simulink model "valve_map"  (R2024b)
settings: Solver=FixedStepDiscrete  StartTime=0.0  StopTime=300  FixedStep=dev.dt  RelTol=1e-3
undefined symbols (not defined in the file or in its folder): disfilt, dspblkCoreblockFVToolHelper, dt, gcbh
libraries: simulink x1, subsignallib x1
settings Model: SimulationMode=external  ExtModeEnableFloating=off  ExtModeTrigDuration=100000  Creator=pro  LastModifiedBy=af49v
settings SolverCC: ConcurrentTasks=on  AlgebraicLoopSolver=TrustRegion  PositivePriorityOrder=on  AutoInsertRateTranBlk=on
settings DataIOCC: MaxDataPoints=500  SaveOutput=off  DSMLogging=off  SaveTime=off  ReturnWorkspaceOutputs=off
settings OptimizationCC: BlockReduction=off  OptimizeBlockIOStorage=off  EnhancedBackFolding=on  PassReuseOutputArgsThreshold=0  MaxStackSize=64  OptimizeBlockOrder=speed  DifferentSizesBufferReuse=on
settings DebuggingCC: AlgebraicLoopMsg=error  TasksWithSamePriorityMsg=none  IntegerOverflowMsg=error  ParameterUnderflowMsg=error  ParameterTunabilityLossMsg=error  UnconnectedInputMsg=warning  UnconnectedOutputMsg=warning  UnconnectedLineMsg=warning  AllowSymbolicDim=off  NonBusSignalsTreatedAsBus=error  SFInvalidInputDataAccessInChartInitDiag=error
settings HardwareCC: ProdBitPerLong=64  ProdLongLongMode=on  ProdHWDeviceType=Intel->x86-64 (Linux 64)  HardwareBoardFeatureSet=SoCBlockset
settings ModelReferenceCC: EnableRefExpFcnMdlSchedulingChecks=on
settings SFSimCC: MATLABDynamicMemAlloc=off
settings RTWCC: Description=Speedgoat Real-Time Target Machine  SystemTargetFile=speedgoat.tlc  TemplateMakefile=slrealtime_default_tmf  RTWVerbose=off  Toolchain=Simulink Real-Time Toolchain  BuildConfiguration=Faster Runs  CodeExecutionProfiling=on  TargetLang=C++  GPUComputeCapability=3.5  DLArmComputeVersion=19.05
settings CodeAppCC: ForceParamTrailComments=on  OperatorAnnotations=on
settings SimulinkRealTimeTargetCC: InstructionSetFMA=off  LogToMDFFile=off

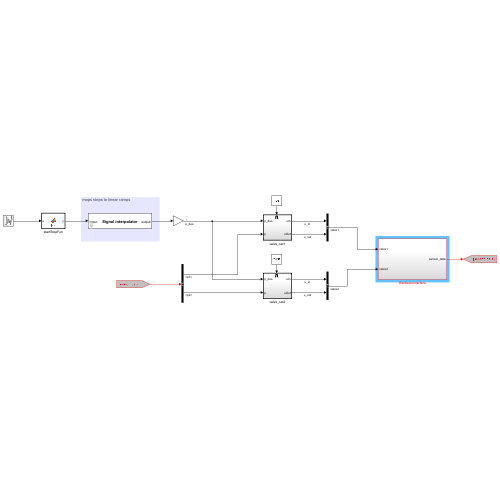
[thumbnail: Simulink's stored preview of the top-level diagram]
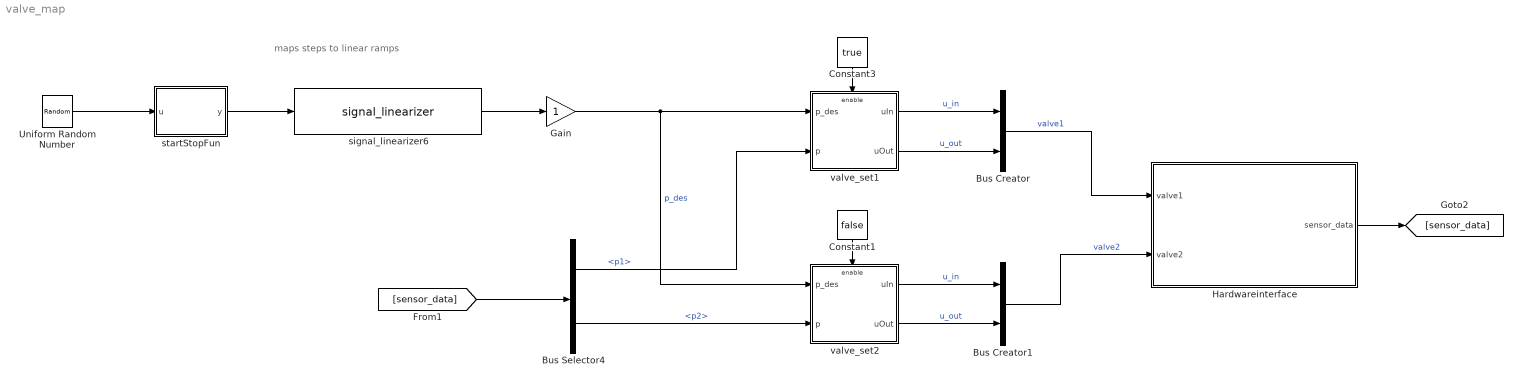
== system valve_map ==
  note: maps steps to linear ramps
  Bus Creator : BusCreator  Inputs=2
  Bus Creator1 : BusCreator  Inputs=2
  Bus Selector4 : BusSelector  OutputSignals=p1,p2
  Constant1 : Constant  Value=false
  Constant3 : Constant  Value=true
  Gain : Gain
  Hardwareinterface : Subsystem
  Uniform Random Number : UniformRandomNumber  Minimum=-0.5  Maximum=6.5  SampleTime=dt
  signal_linearizer6 : subsignallib/signal_linearizer  param_low=1  param_high=dt  es_filt_enabled=on  es_ts=4
      settings: SourceProductName=Signals
  startStopFun : MATLAB Function  TreatAsAtomicUnit=on
  valve_set1 : Subsystem
  valve_set2 : Subsystem
  wires:
  Bus Selector4/1 -> valve_set1/2(p)  "<p1>"
  Gain/1 -> valve_set1/1(p_des), valve_set2/1(p_des)  "p_des"
  Bus Selector4/2 -> valve_set2/2(p)  "<p2>"
  valve_set1/2(uOut) -> Bus Creator/2  "u_out"
  Constant1/1 -> valve_set2/Enable
  Constant3/1 -> valve_set1/Enable
  startStopFun/1(y) -> signal_linearizer6/1
  signal_linearizer6/1 -> Gain/1
  Uniform Random Number/1 -> startStopFun/1(u)
  valve_set2/1(uIn) -> Bus Creator1/1  "u_in"
  valve_set1/1(uIn) -> Bus Creator/1  "u_in"
  [sensor_data] -> Bus Selector4/1
  Bus Creator1/1 -> Hardwareinterface/2(valve2)  "valve2"
  Bus Creator/1 -> Hardwareinterface/1(valve1)  "valve1"
  Hardwareinterface/1(sensor_data) -> [sensor_data]
  valve_set2/2(uOut) -> Bus Creator1/2  "u_out"

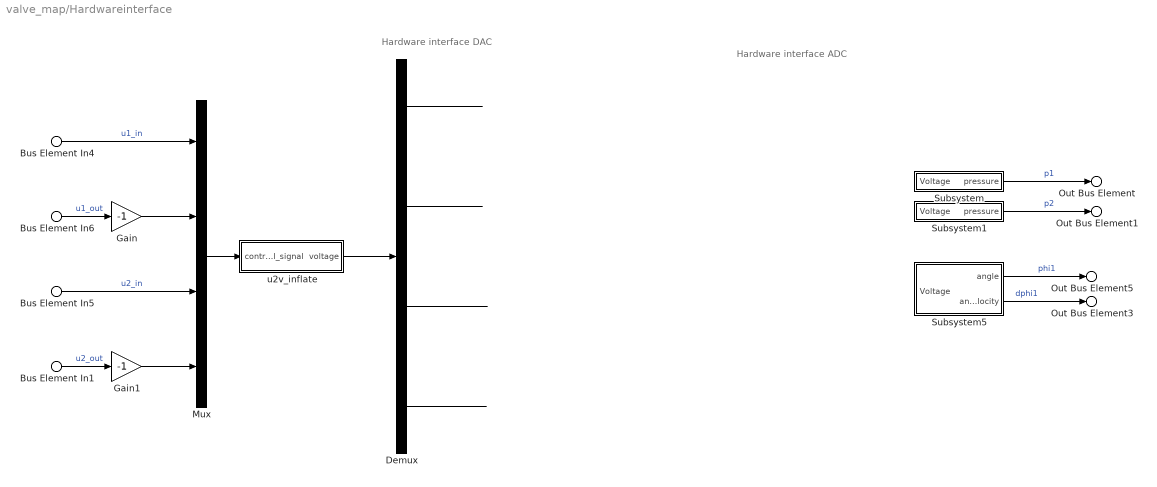
== system valve_map/Hardwareinterface ==
  note: Hardware interface ADC
  note: Hardware interface DAC
  Bus Element In4 : Inport  PortName=valve1  Element=u_in
  Bus Element In6 : Inport  PortName=valve1  Element=u_out
  Bus Element In5 : Inport  Port=2  PortName=valve2  Element=u_in
  Bus Element In1 : Inport  Port=2  PortName=valve2  Element=u_out
  Demux : Demux
  Gain : Gain  Gain=-1
  Gain1 : Gain  Gain=-1
  Mux : Mux
  Subsystem : Subsystem
  Subsystem1 : Subsystem
  Subsystem5 : Subsystem
  u2v_inflate : Subsystem
  Out Bus Element : Outport  PortName=sensor_data  Element=p1
  Out Bus Element1 : Outport  PortName=sensor_data  Element=p2
  Out Bus Element5 : Outport  PortName=sensor_data  Element=phi1
  Out Bus Element3 : Outport  PortName=sensor_data  Element=dphi1
  wires:
  Subsystem/1(pressure) -> Out Bus Element/1  "p1"
  ? -> Subsystem/1(Voltage)
  ? -> Subsystem1/1(Voltage)
  Subsystem1/1(pressure) -> Out Bus Element1/1  "p2"
  Bus Element In4/1 -> Mux/1  "u1_in"
  ? -> Subsystem5/1(Voltage)
  Subsystem5/1(angle) -> Out Bus Element5/1  "phi1"
  Bus Element In6/1 -> Gain/1  "u1_out"
  Gain/1 -> Mux/2
  Bus Element In5/1 -> Mux/3  "u2_in"
  Bus Element In1/1 -> Gain1/1  "u2_out"
  Gain1/1 -> Mux/4
  Subsystem5/2(angle velocity) -> Out Bus Element3/1  "dphi1"
  Mux/1 -> u2v_inflate/1(control_signal)
  u2v_inflate/1(voltage) -> Demux/1
  Demux/1 -> ?
  Demux/2 -> ?
  Demux/3 -> ?
  Demux/4 -> ?

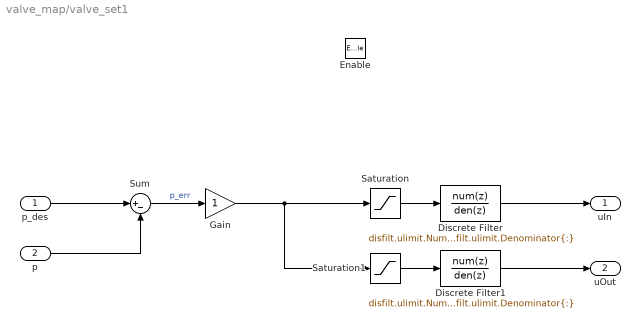
== system valve_map/valve_set1 ==
  p_des : Inport
  p : Inport  Port=2
  Enable : EnablePort
  Discrete Filter : DiscreteFilter  LoadFcn=dspblkCoreblockFVToolHelper(gcbh,'load');  Numerator=disfilt.ulimit.Numerator{:}  Denominator=disfilt.ulimit.Denominator{:}  InitialStates=0.2
      settings: CopyFcn=dspblkCoreblockFVToolHelper(gcbh,'copy');  DeleteFcn=dspblkCoreblockFVToolHelper(gcbh,'close');  ModelCloseFcn=dspblkCoreblockFVToolHelper(gcbh,'close');  PreSaveFcn=dspblkCoreblockFVToolHelper(gcbh,'presave');  PostSaveFcn=dspblkCoreblockFVToolHelper(gcbh,'postsave');  CloseFcn=dspblkCoreblockFVToolHelper(gcbh,'close');
  Discrete Filter1 : DiscreteFilter  LoadFcn=dspblkCoreblockFVToolHelper(gcbh,'load');  Numerator=disfilt.ulimit.Numerator{:}  Denominator=disfilt.ulimit.Denominator{:}  InitialStates=-0.2
      settings: CopyFcn=dspblkCoreblockFVToolHelper(gcbh,'copy');  DeleteFcn=dspblkCoreblockFVToolHelper(gcbh,'close');  ModelCloseFcn=dspblkCoreblockFVToolHelper(gcbh,'close');  PreSaveFcn=dspblkCoreblockFVToolHelper(gcbh,'presave');  PostSaveFcn=dspblkCoreblockFVToolHelper(gcbh,'postsave');  CloseFcn=dspblkCoreblockFVToolHelper(gcbh,'close');
  Gain : Gain
  Saturation : Saturate  UpperLimit=1  LowerLimit=0
  Saturation1 : Saturate  UpperLimit=0  LowerLimit=-1
  Sum : Sum  Inputs=|+-
  uIn : Outport  OutputWhenDisabled=reset  InitialOutput=0
  uOut : Outport  Port=2  OutputWhenDisabled=reset  InitialOutput=0
  wires:
  Gain/1 -> Saturation/1, Saturation1/1
  Sum/1 -> Gain/1  "p_err"
  p/1 -> Sum/2
  p_des/1 -> Sum/1
  Saturation1/1 -> Discrete Filter1/1
  Saturation/1 -> Discrete Filter/1
  Discrete Filter/1 -> uIn/1
  Discrete Filter1/1 -> uOut/1

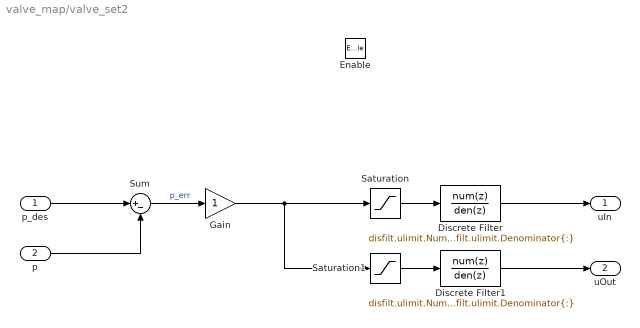
== system valve_map/valve_set2 ==
  p_des : Inport
  p : Inport  Port=2
  Enable : EnablePort
  Discrete Filter : DiscreteFilter  LoadFcn=dspblkCoreblockFVToolHelper(gcbh,'load');  Numerator=disfilt.ulimit.Numerator{:}  Denominator=disfilt.ulimit.Denominator{:}  InitialStates=0.2
      settings: CopyFcn=dspblkCoreblockFVToolHelper(gcbh,'copy');  DeleteFcn=dspblkCoreblockFVToolHelper(gcbh,'close');  ModelCloseFcn=dspblkCoreblockFVToolHelper(gcbh,'close');  PreSaveFcn=dspblkCoreblockFVToolHelper(gcbh,'presave');  PostSaveFcn=dspblkCoreblockFVToolHelper(gcbh,'postsave');  CloseFcn=dspblkCoreblockFVToolHelper(gcbh,'close');
  Discrete Filter1 : DiscreteFilter  LoadFcn=dspblkCoreblockFVToolHelper(gcbh,'load');  Numerator=disfilt.ulimit.Numerator{:}  Denominator=disfilt.ulimit.Denominator{:}  InitialStates=-0.2
      settings: CopyFcn=dspblkCoreblockFVToolHelper(gcbh,'copy');  DeleteFcn=dspblkCoreblockFVToolHelper(gcbh,'close');  ModelCloseFcn=dspblkCoreblockFVToolHelper(gcbh,'close');  PreSaveFcn=dspblkCoreblockFVToolHelper(gcbh,'presave');  PostSaveFcn=dspblkCoreblockFVToolHelper(gcbh,'postsave');  CloseFcn=dspblkCoreblockFVToolHelper(gcbh,'close');
  Gain : Gain
  Saturation : Saturate  UpperLimit=1  LowerLimit=0
  Saturation1 : Saturate  UpperLimit=0  LowerLimit=-1
  Sum : Sum  Inputs=|+-
  uIn : Outport  OutputWhenDisabled=reset  InitialOutput=0
  uOut : Outport  Port=2  OutputWhenDisabled=reset  InitialOutput=0
  wires:
  Gain/1 -> Saturation/1, Saturation1/1
  Sum/1 -> Gain/1  "p_err"
  p/1 -> Sum/2
  p_des/1 -> Sum/1
  Saturation1/1 -> Discrete Filter1/1
  Saturation/1 -> Discrete Filter/1
  Discrete Filter/1 -> uIn/1
  Discrete Filter1/1 -> uOut/1

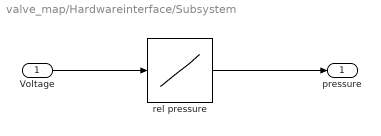
== system valve_map/Hardwareinterface/Subsystem ==
  Voltage : Inport
  rel pressure : Lookup_n-D  NumberOfTableDimensions=1  BreakpointsForDimension1=[0 10]  Table=[0 10]  InternalRulePriority=Speed  RndMeth=Simplest
  pressure : Outport  VectorParamsAs1DForOutWhenUnconnected=off
  wires:
  Voltage/1 -> rel pressure/1
  rel pressure/1 -> pressure/1

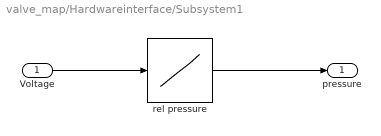
== system valve_map/Hardwareinterface/Subsystem1 ==
  Voltage : Inport
  rel pressure : Lookup_n-D  NumberOfTableDimensions=1  BreakpointsForDimension1=[0 10]  Table=[0 10]  InternalRulePriority=Speed  RndMeth=Simplest
  pressure : Outport  VectorParamsAs1DForOutWhenUnconnected=off
  wires:
  Voltage/1 -> rel pressure/1
  rel pressure/1 -> pressure/1

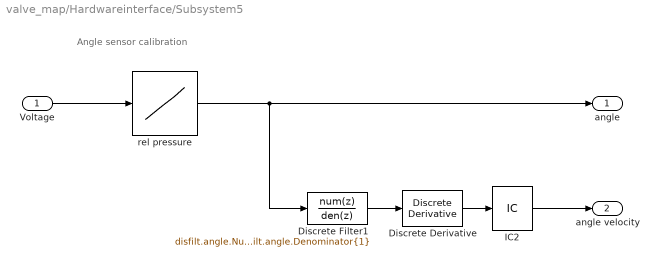
== system valve_map/Hardwareinterface/Subsystem5 ==
  note: Angle sensor calibration
  Voltage : Inport
  Discrete Derivative : simulink/Discrete/Discrete Derivative  gainval=1.0  ICPrevScaledInput=0.0  OutMin=[]  OutMax=[]  OutDataType=fixdt(1, 16)  OutScaling=2^-10  DoSatur=off
  Discrete Filter1 : DiscreteFilter  LoadFcn=dspblkCoreblockFVToolHelper(gcbh,'load');  Numerator=disfilt.angle.Numerator{1}  Denominator=disfilt.angle.Denominator{1}
      settings: CopyFcn=dspblkCoreblockFVToolHelper(gcbh,'copy');  DeleteFcn=dspblkCoreblockFVToolHelper(gcbh,'close');  ModelCloseFcn=dspblkCoreblockFVToolHelper(gcbh,'close');  PreSaveFcn=dspblkCoreblockFVToolHelper(gcbh,'presave');  PostSaveFcn=dspblkCoreblockFVToolHelper(gcbh,'postsave');  CloseFcn=dspblkCoreblockFVToolHelper(gcbh,'close');
  IC2 : InitialCondition
  rel pressure : Lookup_n-D  NumberOfTableDimensions=1  BreakpointsForDimension1=[2.167 3.14]  Table=[0.7854 -0.7854]  InternalRulePriority=Speed  RndMeth=Simplest
  angle : Outport  VectorParamsAs1DForOutWhenUnconnected=off
  angle velocity : Outport  Port=2  VectorParamsAs1DForOutWhenUnconnected=off
  wires:
  Discrete Derivative/1 -> IC2/1
  IC2/1 -> angle velocity/1
  rel pressure/1 -> angle/1, Discrete Filter1/1
  Discrete Filter1/1 -> Discrete Derivative/1
  Voltage/1 -> rel pressure/1

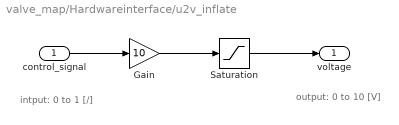
== system valve_map/Hardwareinterface/u2v_inflate ==
  note: intput: 0 to 1 [/]
  note: output: 0 to 10 [V]
  control_signal : Inport
  Gain : Gain  Gain=10
  Saturation : Saturate  UpperLimit=10  LowerLimit=0
  voltage : Outport  VectorParamsAs1DForOutWhenUnconnected=off
  wires:
  Gain/1 -> Saturation/1
  control_signal/1 -> Gain/1
  Saturation/1 -> voltage/1

== matlab function valve_map/startStopFun ==
  data: u input; y output
function y = fcn(u)
y = 0;
persistent t
if isempty(t)
    t = 0; % wait n samples
    return
end
t = t+1;
dt = 0.005;
tStart = 2/dt;
tEnd = 290/dt;

if t > tStart && t < tEnd
    y = u;
else
    y = 0;
end
